simulink subsystem "RRR_rigid_joints"  (R2021b)
settings: Solver=VariableStepAuto  StartTime=0.0  StopTime=10.0  RelTol=1e-3
undefined symbols (not defined in the file): dq0, friction, q0
settings Model: Creator=fabioscap  LastModifiedBy=fabioscap

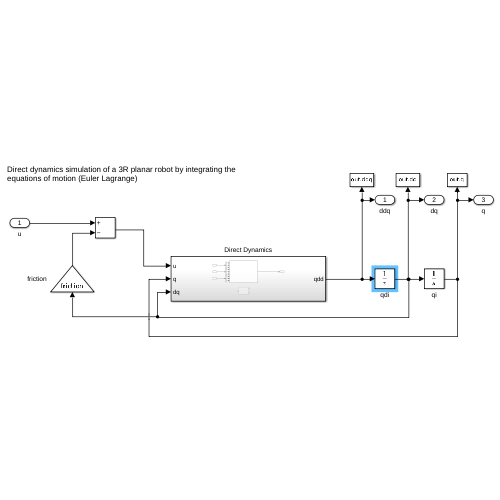
[thumbnail: Simulink's stored preview of the top-level diagram]
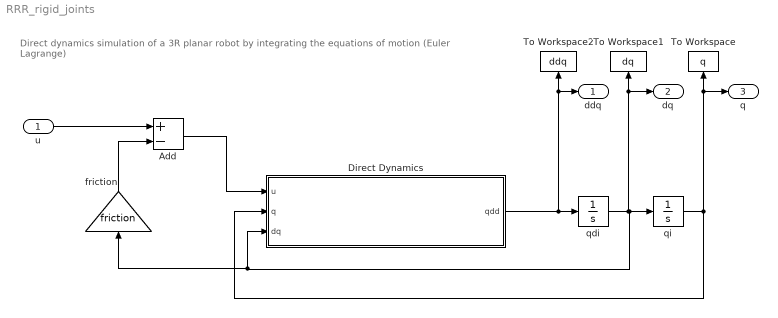
== system RRR_rigid_joints ==
  note: Direct dynamics simulation of a 3R planar robot by integrating the equations of motion (Euler Lagrange)
  u : Inport  PortDimensions=3
  Add : Sum  Inputs=+-
  Direct Dynamics : Subsystem
  To Workspace : ToWorkspace  VariableName=q  SaveFormat=Timeseries  SampleTime=-1
  To Workspace1 : ToWorkspace  VariableName=dq  SaveFormat=Timeseries  SampleTime=-1
  To Workspace2 : ToWorkspace  VariableName=ddq  SaveFormat=Timeseries  SampleTime=-1
  friction : Gain  Gain=friction
  qdi : Integrator  InitialCondition=dq0
  qi : Integrator  InitialCondition=q0
  ddq : Outport  PortDimensions=3
  dq : Outport  Port=2  PortDimensions=3
  q : Outport  Port=3  PortDimensions=3
  wires:
  u/1 -> Add/1
  friction/1 -> Add/2
  qdi/1 -> friction/1, Direct Dynamics/3(dq), qi/1, dq/1, To Workspace1/1
  Direct Dynamics/1(qdd) -> ddq/1, To Workspace2/1, qdi/1
  Add/1 -> Direct Dynamics/1(u)
  qi/1 -> q/1, To Workspace/1, Direct Dynamics/2(q)

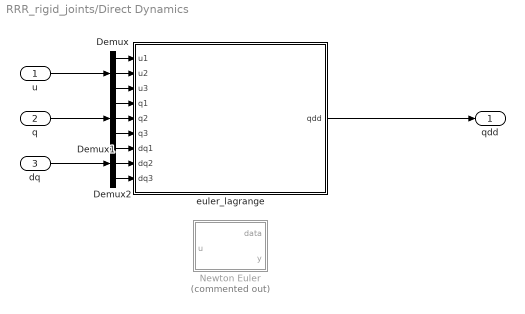
== system RRR_rigid_joints/Direct Dynamics ==
  u : Inport
  q : Inport  Port=2
  dq : Inport  Port=3
  Demux : Demux  Outputs=3
  Demux1 : Demux  Outputs=3
  Demux2 : Demux  Outputs=3
  Newton Euler : MATLAB Function  Commented=on  TreatAsAtomicUnit=on
  euler_lagrange : MATLAB Function  TreatAsAtomicUnit=on
  qdd : Outport
  wires:
  Demux1/1 -> euler_lagrange/4(q1)
  Demux2/1 -> euler_lagrange/7(dq1)
  Demux2/3 -> euler_lagrange/9(dq3)
  Demux/2 -> euler_lagrange/2(u2)
  Demux/1 -> euler_lagrange/1(u1)
  Demux1/3 -> euler_lagrange/6(q3)
  q/1 -> Demux1/1
  Demux2/2 -> euler_lagrange/8(dq2)
  u/1 -> Demux/1
  Demux1/2 -> euler_lagrange/5(q2)
  dq/1 -> Demux2/1
  euler_lagrange/1(qdd) -> qdd/1
  Demux/3 -> euler_lagrange/3(u3)

== matlab function RRR_rigid_joints/Direct Dynamics/euler_lagrange ==
  data: u1 input; qdd output; u2 input; u3 input; q1 input; q2 input; q3 input; dq1 input; dq2 input; dq3 input
function qdd = euler_lagrange(u1,u2,u3,q1,q2,q3,dq1,dq2,dq3)
%#codegen

%    This function was generated by the Symbolic Math Toolbox version 9.0.
%    22-Jul-2022 20:00:41

t2 = cos(q1);
t3 = cos(q2);
t4 = cos(q3);
t5 = sin(q1);
t6 = sin(q2);
t7 = sin(q3);
t8 = q2+q3;
t9 = dq1.^2;
t10 = dq2.^2;
t11 = dq3.^2;
t23 = u1.*8.0e+2;
t12 = t3.^2;
t13 = t3.^3;
t14 = t4.^2;
t15 = t4.^3;
t16 = t7.^2;
t17 = t7.^3;
t18 = cos(t8);
t19 = sin(t8);
t27 = t2.*1.962e+4;
t30 = t3.*u1.*1.2e+3;
t31 = t3.*u2.*1.2e+3;
t32 = t3.*u3.*1.2e+3;
t33 = dq1.*dq2.*t6.*2.4e+3;
t34 = dq1.*dq3.*t7.*3.2e+3;
t35 = dq2.*dq3.*t7.*3.2e+3;
t39 = t6.*t10.*1.2e+3;
t40 = t7.*t11.*1.6e+3;
t41 = t2.*t3.*1.7658e+4;
t48 = t5.*t6.*4.7088e+4;
t50 = t3.*t4.*u3.*1.8e+3;
t64 = dq1.*dq2.*t3.*t7.*1.2e+3;
t65 = dq1.*dq3.*t3.*t7.*1.2e+3;
t66 = dq2.*dq3.*t3.*t7.*1.2e+3;
t67 = dq1.*dq2.*t3.*t6.*3.6e+3;
t80 = t3.*t7.*t9.*6.0e+2;
t81 = t3.*t7.*t10.*6.0e+2;
t82 = t3.*t7.*t11.*6.0e+2;
t83 = t3.*t6.*t9.*1.8e+3;
t84 = t3.*t6.*t10.*1.8e+3;
t89 = t3.*t5.*t6.*1.7658e+4;
t102 = dq1.*dq2.*t3.*t4.*t7.*1.8e+3;
t123 = t3.*t4.*t7.*t9.*9.0e+2;
t124 = t3.*t4.*t7.*t10.*9.0e+2;
t128 = t2.*t4.*t6.*t7.*2.3544e+4;
t129 = t3.*t4.*t5.*t7.*2.3544e+4;
t191 = t2.*t3.*t4.*t6.*t7.*8.829e+3;
t20 = t18.^2;
t21 = t19.^2;
t22 = t19.^3;
t24 = t12.*9.0;
t25 = t14.*1.2e+1;
t26 = t16.*4.8e+1;
t36 = -t27;
t38 = -t31;
t42 = t14.*u1.*6.0e+2;
t43 = t14.*u2.*6.0e+2;
t44 = -t34;
t45 = -t35;
t46 = t16.*u1.*2.4e+3;
t47 = t16.*u2.*2.4e+3;
t49 = t18.*u3.*1.2e+3;
t51 = -t40;
t54 = -t48;
t56 = t3.*t4.*t18.*9.0;
t57 = t3.*t7.*t19.*3.6e+1;
t58 = t9.*t19.*4.0e+2;
t59 = t10.*t19.*4.0e+2;
t60 = t11.*t19.*4.0e+2;
t61 = dq1.*dq2.*t19.*8.0e+2;
t62 = dq1.*dq3.*t19.*8.0e+2;
t63 = dq2.*dq3.*t19.*8.0e+2;
t68 = t4.*t18.*u1.*6.0e+2;
t69 = t4.*t18.*u2.*6.0e+2;
t70 = t4.*t18.*u3.*6.0e+2;
t71 = t2.*t14.*1.4715e+4;
t72 = t2.*t12.*1.7658e+4;
t73 = t7.*t19.*u1.*2.4e+3;
t74 = t7.*t19.*u2.*2.4e+3;
t75 = t7.*t19.*u3.*2.4e+3;
t76 = t2.*t16.*5.886e+4;
t85 = -t64;
t86 = -t65;
t87 = -t66;
t90 = dq1.*dq2.*t6.*t14.*1.8e+3;
t92 = dq1.*dq2.*t6.*t16.*7.2e+3;
t98 = dq1.*dq2.*t3.*t19.*1.2e+3;
t99 = dq1.*dq2.*t7.*t18.*1.2e+3;
t100 = dq1.*dq3.*t3.*t19.*1.2e+3;
t101 = dq2.*dq3.*t3.*t19.*1.2e+3;
t104 = -t80;
t105 = -t81;
t106 = -t82;
t108 = -t89;
t109 = t6.*t9.*t14.*9.0e+2;
t110 = t6.*t10.*t14.*9.0e+2;
t111 = t2.*t3.*t14.*2.3544e+4;
t112 = t4.*t7.*t19.*u3.*3.6e+3;
t113 = t6.*t9.*t16.*3.6e+3;
t114 = t6.*t10.*t16.*3.6e+3;
t115 = t5.*t6.*t14.*2.3544e+4;
t116 = t3.*t9.*t19.*6.0e+2;
t117 = t7.*t9.*t18.*6.0e+2;
t118 = t3.*t10.*t19.*6.0e+2;
t119 = t7.*t10.*t18.*6.0e+2;
t120 = t3.*t11.*t19.*6.0e+2;
t121 = t4.*t9.*t19.*2.4e+3;
t122 = t2.*t4.*t18.*1.4715e+4;
t125 = -t102;
t126 = t16.*t18.*u3.*3.6e+3;
t127 = t2.*t7.*t19.*5.886e+4;
t130 = t9.*t14.*t19.*3.0e+2;
t131 = t10.*t14.*t19.*3.0e+2;
t132 = t11.*t14.*t19.*3.0e+2;
t134 = dq1.*dq2.*t14.*t19.*6.0e+2;
t135 = dq1.*dq3.*t14.*t19.*6.0e+2;
t137 = dq2.*dq3.*t14.*t19.*6.0e+2;
t139 = dq1.*dq2.*t17.*t18.*3.6e+3;
t141 = t4.*t7.*t18.*t19.*1.8e+1;
t142 = t4.*t7.*t9.*t18.*3.0e+2;
t143 = t4.*t7.*t10.*t18.*3.0e+2;
t144 = t4.*t7.*t11.*t18.*3.0e+2;
t145 = dq1.*dq2.*t4.*t7.*t18.*6.0e+2;
t146 = dq1.*dq3.*t4.*t7.*t18.*6.0e+2;
t147 = dq2.*dq3.*t4.*t7.*t18.*6.0e+2;
t148 = dq1.*dq2.*t4.*t6.*t18.*1.8e+3;
t149 = t2.*t6.*t7.*t18.*5.886e+3;
t150 = t3.*t5.*t7.*t18.*5.886e+3;
t151 = dq1.*dq2.*t6.*t7.*t19.*7.2e+3;
t154 = -t123;
t155 = -t124;
t160 = t9.*t17.*t18.*1.8e+3;
t162 = t10.*t17.*t18.*1.8e+3;
t169 = t3.*t5.*t6.*t14.*8.829e+3;
t170 = t4.*t5.*t7.*t12.*8.829e+3;
t173 = t9.*t18.*t19.*6.0e+2;
t177 = t4.*t6.*t9.*t18.*9.0e+2;
t178 = t3.*t4.*t9.*t19.*9.0e+2;
t179 = t4.*t6.*t10.*t18.*9.0e+2;
t184 = t2.*t12.*t14.*8.829e+3;
t185 = t6.*t7.*t9.*t19.*3.6e+3;
t186 = t6.*t7.*t10.*t19.*3.6e+3;
t189 = t4.*t5.*t6.*t18.*1.4715e+4;
t190 = t2.*t3.*t7.*t19.*3.5316e+4;
t192 = t5.*t6.*t7.*t19.*3.5316e+4;
t196 = t4.*t9.*t18.*t19.*3.0e+2;
t197 = t4.*t10.*t18.*t19.*3.0e+2;
t198 = t4.*t11.*t18.*t19.*3.0e+2;
t199 = dq1.*dq2.*t4.*t18.*t19.*6.0e+2;
t200 = dq1.*dq3.*t4.*t18.*t19.*6.0e+2;
t201 = dq2.*dq3.*t4.*t18.*t19.*6.0e+2;
t206 = dq1.*dq2.*t4.*t16.*t19.*3.6e+3;
t208 = t5.*t7.*t12.*t18.*8.829e+3;
t209 = t2.*t6.*t17.*t18.*1.7658e+4;
t210 = t3.*t5.*t17.*t18.*1.7658e+4;
t211 = t3.*t9.*t18.*t19.*9.0e+2;
t212 = t2.*t3.*t6.*t7.*t18.*8.829e+3;
t213 = t3.*t4.*t5.*t6.*t18.*8.829e+3;
t214 = t2.*t4.*t12.*t18.*8.829e+3;
t215 = t4.*t9.*t16.*t19.*1.8e+3;
t217 = t4.*t10.*t16.*t19.*1.8e+3;
t226 = dq1.*dq2.*t16.*t18.*t19.*3.6e+3;
t233 = t9.*t16.*t18.*t19.*1.8e+3;
t235 = t10.*t16.*t18.*t19.*1.8e+3;
t236 = t4.*t16.*t18.*t41;
t237 = t7.*t14.*t19.*t41;
t238 = t4.*t5.*t6.*t16.*t18.*1.7658e+4;
t239 = t2.*t4.*t6.*t16.*t19.*1.7658e+4;
t240 = t3.*t4.*t5.*t16.*t19.*1.7658e+4;
t243 = t5.*t6.*t7.*t14.*t19.*1.7658e+4;
t245 = t2.*t3.*t7.*t14.*t19.*-1.7658e+4;
t247 = t4.*t7.*t18.*t19.*t41;
t248 = t4.*t5.*t6.*t7.*t18.*t19.*1.7658e+4;
t249 = t2.*t6.*t16.*t18.*t19.*1.7658e+4;
t250 = t3.*t5.*t16.*t18.*t19.*1.7658e+4;
t28 = t20.*3.0;
t29 = -t24;
t37 = t21.*1.2e+1;
t52 = -t43;
t53 = -t47;
t55 = -t49;
t77 = -t56;
t78 = -t57;
t79 = t20.*u2.*6.0e+2;
t88 = t21.*u2.*2.4e+3;
t91 = -t69;
t93 = -t71;
t94 = -t74;
t95 = -t76;
t96 = t16.*t20.*9.0;
t97 = t14.*t21.*9.0;
t133 = t7.*t11.*t20.*3.0e+2;
t136 = dq1.*dq3.*t7.*t20.*6.0e+2;
t138 = dq2.*dq3.*t7.*t20.*6.0e+2;
t140 = -t111;
t152 = -t121;
t153 = -t122;
t156 = -t126;
t157 = -t127;
t159 = t6.*t9.*t20.*9.0e+2;
t161 = t4.*t9.*t22.*1.8e+3;
t163 = t2.*t3.*t20.*8.829e+3;
t166 = t6.*t9.*t21.*3.6e+3;
t167 = t2.*t3.*t21.*3.5316e+4;
t168 = t5.*t6.*t20.*8.829e+3;
t171 = t5.*t6.*t21.*3.5316e+4;
t172 = -t141;
t174 = -t142;
t175 = -t143;
t176 = -t144;
t180 = t3.*t122;
t181 = -t145;
t182 = -t146;
t183 = -t147;
t187 = -t149;
t188 = -t150;
t202 = -t178;
t203 = -t184;
t204 = -t189;
t205 = -t192;
t207 = dq1.*dq2.*t4.*t7.*t21.*3.6e+3;
t216 = t4.*t7.*t9.*t21.*1.8e+3;
t218 = t4.*t7.*t10.*t21.*1.8e+3;
t219 = -t206;
t221 = -t208;
t222 = -t209;
t223 = -t210;
t224 = -t212;
t225 = -t213;
t227 = -t215;
t229 = -t217;
t231 = t14.*t21.*t41;
t232 = t5.*t6.*t14.*t21.*1.7658e+4;
t234 = t7.*t9.*t18.*t21.*1.8e+3;
t241 = t2.*t4.*t6.*t7.*t21.*1.7658e+4;
t242 = t3.*t4.*t5.*t7.*t21.*1.7658e+4;
t244 = t2.*t3.*t14.*t21.*-1.7658e+4;
t246 = -t238;
t251 = -t248;
t252 = -t249;
t253 = -t250;
t103 = -t79;
t107 = -t88;
t158 = -t133;
t164 = -t136;
t165 = -t138;
t193 = -t161;
t194 = -t168;
t195 = -t171;
t220 = -t207;
t228 = -t216;
t230 = -t218;
t254 = t25+t26+t28+t29+t37+t77+t78+t96+t97+t172+1.6e+1;
t255 = 1.0./t254;
et1 = t23+t30+t32+t33+t36+t39+t41+t42+t44+t45+t46+t50+t51+t52+t53+t54+t55+t58+t59+t60+t61+t62+t63+t67+t68+t70+t72+t73+t75+t84+t85+t86+t87+t90+t92+t93+t95+t98+t99+t100+t101+t103+t104+t105+t106+t107+t108+t109+t110+t112+t113+t114+t115+t116+t117+t118+t119+t120+t125+t128+t129+t130+t131+t132+t134+t135+t137+t139+t140+t148+t151+t152+t153+t154+t155+t156+t157+t158+t159+t160+t162+t163+t164+t165+t166+t167+t169+t170+t173+t174+t175+t176+t179+t180+t181+t182+t183+t186+t187+t188+t190+t191+t193+t194+t195+t196+t197+t198+t199+t200+t201+t202+t203+t204+t205+t211+t214+t219+t220+t221+t222+t223+t224+t225+t226+t227+t229+t230+t232+t234+t235+t236+t239+t240+t241+t242+t243+t244+t245+t246+t247+t251+t252+t253-u2.*4.0e+3+u3.*3.2e+3+t6.*t9.*6.0e+3-t7.*t9.*1.6e+3-t7.*t10.*1.6e+3-t3.*u2.*2.4e+3+t4.*u3.*4.8e+3;
et2 = t20.*u3.*6.0e+2+t21.*u3.*2.4e+3-dq1.*dq2.*t7.*3.2e+3+t3.*t6.*t9.*3.6e+3-t4.*t7.*t9.*2.4e+3-t4.*t7.*t10.*2.4e+3-t7.*t9.*t20.*3.0e+2-t7.*t10.*t20.*3.0e+2-t3.*t18.*u3.*1.8e+3-t4.*t18.*u2.*1.2e+3+t4.*t21.*u3.*3.6e+3-t7.*t19.*u2.*4.8e+3-dq1.*dq2.*t4.*t7.*4.8e+3-dq1.*dq2.*t7.*t20.*6.0e+2+t3.*t7.*t9.*t18.*9.0e+2+t4.*t6.*t9.*t18.*1.8e+3+t3.*t7.*t10.*t18.*9.0e+2-t4.*t7.*t9.*t21.*3.6e+3+t6.*t7.*t9.*t19.*7.2e+3+t9.*t16.*t18.*t19.*3.6e+3-t7.*t18.*t19.*u3.*3.6e+3+dq1.*dq2.*t3.*t7.*t18.*1.8e+3;
et3 = t30+t38+t41+t44+t45+t51+t54+t67+t68+t73+t83+t84+t91+t94+t98+t100+t101+t103+t107+t115+t116+t118+t120+t128+t129+t140+t148+t151+t152+t153+t157+t158+t159+t163+t164+t165+t166+t167-t173+t177+t178+t179+t185+t186+t193+t194+t195+t196+t197+t198+t199+t200+t201+t211+t214+t220+t221+t224+t225+t226+t228+t230+t232+t233+t234+t235+t241+t242+t244+t247+t251+t252+t253-u2.*3.2e+3+u3.*6.4e+3+t6.*t9.*4.8e+3-t7.*t9.*3.2e+3-t7.*t10.*3.2e+3+t2.*t18.*2.943e+4-t9.*t17.*4.8e+3-t10.*t17.*4.8e+3-t9.*t19.*1.6e+3-t9.*t22.*1.2e+3+t15.*t48+t15.*t171-t4.*u2.*4.8e+3+t4.*u3.*9.6e+3-t12.*u3.*1.8e+3+t14.*u3.*9.6e+3+t16.*u3.*9.6e+3;
et4 = t18.*u1.*-1.2e+3+t18.*u2.*1.2e+3+t20.*u3.*3.0e+3+t21.*u3.*4.8e+3-dq1.*dq2.*t7.*6.4e+3-dq1.*dq2.*t17.*9.6e+3+t2.*t3.*t4.*1.0791e+4+t2.*t6.*t7.*1.5696e+4+t3.*t5.*t7.*1.5696e+4-t4.*t5.*t6.*5.4936e+4+t2.*t4.*t13.*8.829e+3+t4.*t6.*t9.*7.2e+3-t2.*t3.*t15.*4.7088e+4-t4.*t7.*t9.*4.8e+3-t4.*t7.*t10.*4.8e+3-t4.*t7.*t11.*2.4e+3+t2.*t6.*t17.*4.7088e+4+t3.*t5.*t17.*4.7088e+4-t5.*t7.*t13.*8.829e+3+t7.*t9.*t12.*9.0e+2+t7.*t10.*t12.*9.0e+2-t7.*t9.*t14.*4.8e+3;
et5 = t7.*t10.*t14.*-4.8e+3-t2.*t12.*t18.*2.6487e+4-t6.*t9.*t18.*1.8e+3-t6.*t10.*t18.*1.8e+3+t2.*t16.*t18.*8.829e+4-t7.*t9.*t20.*1.5e+3-t7.*t9.*t21.*1.2e+3-t7.*t10.*t20.*1.5e+3-t7.*t10.*t21.*1.2e+3+t9.*t12.*t19.*9.0e+2-t9.*t14.*t19.*4.8e+3-t9.*t16.*t19.*4.8e+3-t9.*t14.*t22.*3.6e+3-t9.*t17.*t20.*3.6e+3-t10.*t17.*t20.*3.6e+3-t10.*t18.*t19.*6.0e+2-t9.*t19.*t20.*1.2e+3-t11.*t18.*t19.*6.0e+2+t4.*t16.*t48+t3.*t4.*u1.*1.8e+3-t3.*t4.*u2.*1.8e+3+t3.*t18.*u2.*1.8e+3;
et6 = t3.*t18.*u3.*-3.6e+3-t4.*t21.*u2.*3.6e+3+t4.*t21.*u3.*7.2e+3-t16.*t18.*u1.*3.6e+3+t16.*t18.*u2.*3.6e+3+t14.*t21.*u3.*7.2e+3+t16.*t20.*u3.*7.2e+3-dq1.*dq2.*t4.*t7.*9.6e+3-dq1.*dq3.*t4.*t7.*4.8e+3-dq2.*dq3.*t4.*t7.*4.8e+3+dq1.*dq2.*t7.*t12.*1.8e+3-dq1.*dq2.*t7.*t14.*9.6e+3-dq1.*dq2.*t6.*t18.*3.6e+3-dq1.*dq2.*t7.*t20.*3.0e+3-dq1.*dq2.*t7.*t21.*2.4e+3-dq1.*dq2.*t17.*t20.*7.2e+3-dq1.*dq2.*t18.*t19.*1.2e+3-dq1.*dq3.*t18.*t19.*1.2e+3-dq2.*dq3.*t18.*t19.*1.2e+3+t3.*t4.*t6.*t9.*2.7e+3+t3.*t4.*t6.*t10.*2.7e+3;
et7 = t2.*t3.*t4.*t16.*-4.7088e+4-t2.*t6.*t7.*t12.*8.829e+3-t4.*t5.*t6.*t12.*8.829e+3-t2.*t3.*t4.*t20.*1.1772e+4+t2.*t6.*t7.*t14.*4.7088e+4+t3.*t5.*t7.*t14.*4.7088e+4+t2.*t3.*t4.*t21.*4.1202e+4-t2.*t4.*t7.*t19.*8.829e+4+t3.*t5.*t6.*t18.*2.6487e+4+t2.*t6.*t7.*t20.*1.1772e+4+t3.*t5.*t7.*t20.*1.1772e+4+t4.*t5.*t6.*t20.*1.1772e+4+t2.*t6.*t7.*t21.*1.1772e+4+t3.*t4.*t10.*t19.*9.0e+2+t3.*t5.*t7.*t21.*1.1772e+4-t3.*t6.*t9.*t18.*2.7e+3-t4.*t5.*t6.*t21.*4.1202e+4+t3.*t4.*t11.*t19.*9.0e+2+t3.*t7.*t9.*t18.*1.8e+3;
et8 = t3.*t7.*t10.*t18.*1.8e+3+t3.*t7.*t11.*t18.*9.0e+2+t3.*t7.*t9.*t21.*3.6e+3+t4.*t6.*t9.*t21.*5.4e+3-t2.*t3.*t15.*t21.*3.5316e+4+t2.*t6.*t17.*t20.*3.5316e+4+t3.*t5.*t17.*t20.*3.5316e+4+t2.*t12.*t14.*t18.*3.5316e+4+t3.*t9.*t16.*t19.*3.6e+3+t3.*t10.*t16.*t19.*3.6e+3-t6.*t9.*t16.*t18.*5.4e+3-t6.*t10.*t16.*t18.*5.4e+3-t7.*t9.*t14.*t21.*3.6e+3-t5.*t12.*t16.*t19.*3.5316e+4-t7.*t10.*t14.*t21.*3.6e+3-t9.*t16.*t19.*t20.*3.6e+3-t3.*t4.*t18.*u3.*7.2e+3+t4.*t7.*t19.*u1.*3.6e+3-t3.*t7.*t19.*u3.*7.2e+3-t4.*t7.*t19.*u2.*3.6e+3;
et9 = t7.*t18.*t19.*u2.*3.6e+3-t7.*t18.*t19.*u3.*7.2e+3+dq1.*dq2.*t3.*t4.*t6.*5.4e+3+dq1.*dq2.*t3.*t4.*t19.*1.8e+3+dq1.*dq3.*t3.*t4.*t19.*1.8e+3+dq1.*dq2.*t3.*t7.*t18.*3.6e+3+dq2.*dq3.*t3.*t4.*t19.*1.8e+3+dq1.*dq3.*t3.*t7.*t18.*1.8e+3+dq2.*dq3.*t3.*t7.*t18.*1.8e+3+dq1.*dq2.*t3.*t16.*t19.*7.2e+3-dq1.*dq2.*t6.*t16.*t18.*1.08e+4-dq1.*dq2.*t7.*t14.*t21.*7.2e+3+t3.*t4.*t7.*t9.*t18.*3.6e+3+t3.*t4.*t7.*t10.*t18.*3.6e+3+t2.*t4.*t7.*t12.*t19.*3.5316e+4-t2.*t3.*t4.*t16.*t20.*3.5316e+4+t4.*t6.*t7.*t9.*t19.*5.4e+3-t2.*t3.*t6.*t16.*t19.*3.5316e+4-t3.*t5.*t6.*t14.*t18.*3.5316e+4;
et10 = t4.*t5.*t7.*t12.*t18.*-3.5316e+4+t4.*t6.*t7.*t10.*t19.*5.4e+3-t2.*t3.*t7.*t18.*t19.*5.2974e+4+t2.*t6.*t7.*t14.*t21.*3.5316e+4+t3.*t5.*t7.*t14.*t21.*3.5316e+4+t4.*t5.*t6.*t16.*t20.*3.5316e+4+t3.*t4.*t9.*t18.*t19.*3.6e+3+t5.*t6.*t7.*t18.*t19.*5.2974e+4+t4.*t7.*t9.*t18.*t21.*7.2e+3-t6.*t7.*t9.*t18.*t19.*5.4e+3+t4.*t9.*t16.*t18.*t19.*7.2e+3+t4.*t10.*t16.*t18.*t19.*7.2e+3-t4.*t7.*t18.*t19.*u3.*1.44e+4-t2.*t3.*t4.*t6.*t7.*t18.*3.5316e+4-t3.*t4.*t5.*t6.*t7.*t19.*3.5316e+4+t2.*t3.*t7.*t14.*t18.*t19.*7.0632e+4-t2.*t4.*t6.*t16.*t18.*t19.*7.0632e+4;
et11 = t3.*t4.*t5.*t16.*t18.*t19.*-7.0632e+4-t5.*t6.*t7.*t14.*t18.*t19.*7.0632e+4+dq1.*dq2.*t3.*t4.*t7.*t18.*7.2e+3+dq1.*dq2.*t4.*t6.*t7.*t19.*1.08e+4+dq1.*dq2.*t4.*t16.*t18.*t19.*1.44e+4;
qdd = [t255.*(t23+t32+t33+t36+t38+t39+t42+t46+t50+t52+t53+t55+t58+t59+t60+t61+t62+t63+t70+t72+t75+t83+t85+t86+t87+t90+t91+t92+t93+t94+t95+t99+t104+t105+t106+t108+t109+t110+t112+t113+t114+t117+t119+t125+t130+t131+t132+t134+t135+t137+t139+t154+t155+t156+t160+t162+t169+t170+t173+t174+t175+t176+t177+t180+t181+t182+t183+t185+t187+t188+t190+t191+t202+t203+t204+t205+t219+t222+t223+t227+t228+t229+t233+t236+t239+t240+t243+t245+t246-u2.*8.0e+2+t6.*t9.*1.2e+3).*(3.0./2.0e+2);t255.*(et1+et2).*(-3.0./2.0e+2);t255.*(et3+et4+et5+et6+et7+et8+et9+et10+et11).*(3.0./2.0e+2)];

== matlab function RRR_rigid_joints/Direct Dynamics/Newton Euler ==
  data: data output; u input; y output
function [data, y]= fcn(u)

y = u;
